simulink model "untitled2"  (R2022a)
settings: Solver=ode45  StartTime=0.0  StopTime=2  MaxStep=1e-5  RelTol=1e-3
settings Model: Creator=Administrator  LastModifiedBy=Administrator

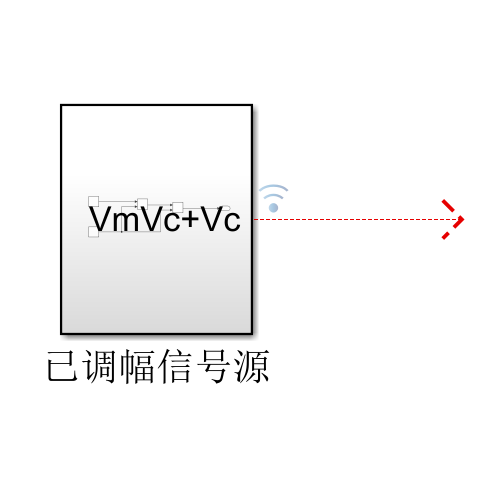
[thumbnail: Simulink's stored preview of the top-level diagram]
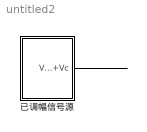
== system untitled2 ==
  已调幅信号源 : Subsystem
  wires:
  已调幅信号源/1(VmVc+Vc) -> ?

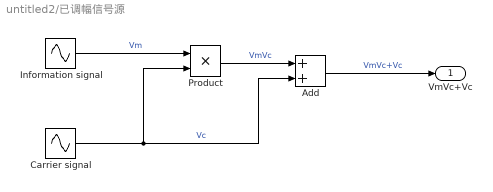
== system untitled2/已调幅信号源 ==
  Add : Sum
  Carrier signal : Sin  Amplitude=1.2  Frequency=1000*2*pi  SampleTime=0
  Information signal : Sin  Amplitude=1.1  Frequency=100*2*pi  SampleTime=0
  Product : Product
  VmVc+Vc : Outport
  wires:
  Information signal/1 -> Product/1  "Vm"
  Carrier signal/1 -> Add/2, Product/2  "Vc"
  Add/1 -> VmVc+Vc/1  "VmVc+Vc"
  Product/1 -> Add/1  "VmVc"
